simulink model "KLTTry"  (R2015a)
settings: Solver=FixedStepDiscrete  StartTime=0.0  StopTime=0.1  FixedStep=0.1  RelTol=1e-3
undefined symbols (not defined in the file or in its folder): fspecial
libraries: visionanalysis x2, visionsources x2
settings Model: CovSFcnEnable=off  Creator=gsalhotr  LastModifiedBy=gsalhotr
settings OptimizationCC: UseDivisionForNetSlopeComputation=Off  SimCompilerOptimization=Off
settings DebuggingCC: SolverPrmCheckMsg=warning  FrameProcessingCompatibilityMsg=warning
settings RTWCC: RTWCompilerOptimization=Off

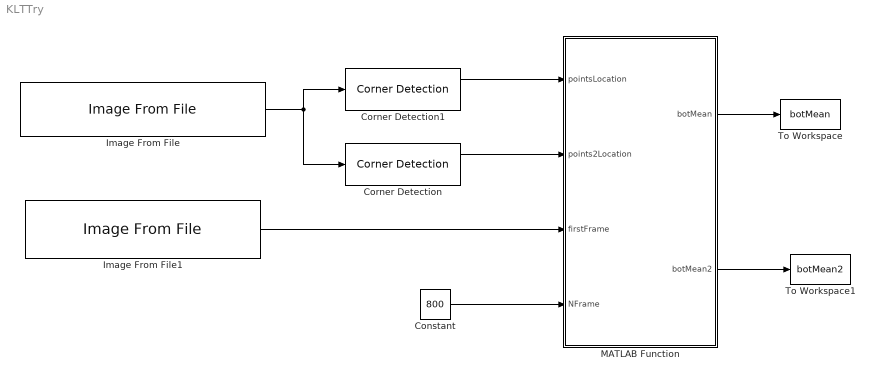
== system KLTTry ==
  Constant : Constant  Value=800
  Corner Detection : visionanalysis/Corner Detection  method=Minimum eigenvalue (Shi & Tomasi)  factor=0.04  filter=fspecial('gaussian', [1 5], 1.5)  thrInten=0.1  thrAngle=157.5  output=Obsolete9b  outputInUse=Corner location  maxNum=50  thrMetric=0.0005  neighborSize=[11 11]  isOutVarDim=off  accumMode=Binary point scaling  accumWordLength=32  accumFracLength=0  prodOutputMode=Binary point scaling  prodOutputWordLength=32  prodOutputFracLength=0  memoryMode=Binary point scaling  memoryWordLength=32  memoryFracLength=0  firstCoeffMode=Specify word length  firstCoeffWordLength=16  firstCoeffFracLength=16  roundingMode=Floor  overflowMode=off
  Corner Detection1 : visionanalysis/Corner Detection  method=Minimum eigenvalue (Shi & Tomasi)  factor=0.04  filter=fspecial('gaussian', [1 5], 1.5)  thrInten=0.1  thrAngle=157.5  output=Obsolete9b  outputInUse=Corner location  maxNum=50  thrMetric=0.0005  neighborSize=[11 11]  isOutVarDim=off  accumMode=Binary point scaling  accumWordLength=32  accumFracLength=0  prodOutputMode=Binary point scaling  prodOutputWordLength=32  prodOutputFracLength=0  memoryMode=Binary point scaling  memoryWordLength=32  memoryFracLength=0  firstCoeffMode=Specify word length  firstCoeffWordLength=16  firstCoeffFracLength=16  roundingMode=Floor  overflowMode=off
  Image From File : visionsources/Image From File  Tag=vipblks_nd  FileName=\\home-00-ah\gsalhotr\Documents\MATLAB\ETRobocon2014Files\Repository\models\host\CVTeam\KLTTracking\media\Lomography1stFrameGray480p.jpg  imagePorts=One multidimensional signal  Ts=inf  ImageDataType=Inherit from input image  Signed=on  WordLength=16  sdImageDataType=uint(8)  FractionLengthMode=User-defined  FractionLength=15  OutPortLabels=R|G|B
  Image From File1 : visionsources/Image From File  Tag=vipblks_nd  FileName=\\home-00-ah\gsalhotr\Documents\MATLAB\ETRobocon2014Files\Repository\models\host\CVTeam\KLTTracking\media\Lomography1stFrame480p.jpg  imagePorts=One multidimensional signal  Ts=inf  ImageDataType=Inherit from input image  Signed=on  WordLength=16  sdImageDataType=uint(8)  FractionLengthMode=User-defined  FractionLength=15  OutPortLabels=R|G|B
  MATLAB Function : MATLAB Function  TreatAsAtomicUnit=on
  To Workspace : ToWorkspace  VariableName=botMean  SaveFormat=Timeseries  SampleTime=-1
  To Workspace1 : ToWorkspace  VariableName=botMean2  SaveFormat=Timeseries  SampleTime=-1
  wires:
  Image From File/1 -> Corner Detection1/1, Corner Detection/1
  Image From File1/1 -> MATLAB Function/3(firstFrame)
  Corner Detection/1 -> MATLAB Function/2(points2Location)
  Corner Detection1/1 -> MATLAB Function/1(pointsLocation)
  Constant/1 -> MATLAB Function/4(NFrame)
  MATLAB Function/1(botMean) -> To Workspace/1
  MATLAB Function/2(botMean2) -> To Workspace1/1

== matlab function KLTTry/MATLAB Function ==
  data: pointsLocation input single size=[50 2]; botMean output; points2Location input; firstFrame input; NFrame input; botMean2 output
function [botMean, botMean2] = fcn(pointsLocation, points2Location, firstFrame, NFrame)
%#codegen
[botMean, botMean2] = KLTTrackerParallel(pointsLocation, points2Location, firstFrame, NFrame);
end
